simulink model "Transferfunction"  (R2021b)
settings: Solver=VariableStepAuto  StartTime=0.0  StopTime=10.0  RelTol=1e-3
libraries: dspsrcs4 x1
settings Model: Creator=Asus  LastModifiedBy=Matina Kaviani
settings SolverCC: AlgebraicLoopSolver=TrustRegion
settings DebuggingCC: SFMachineParentedDataDiag=warning

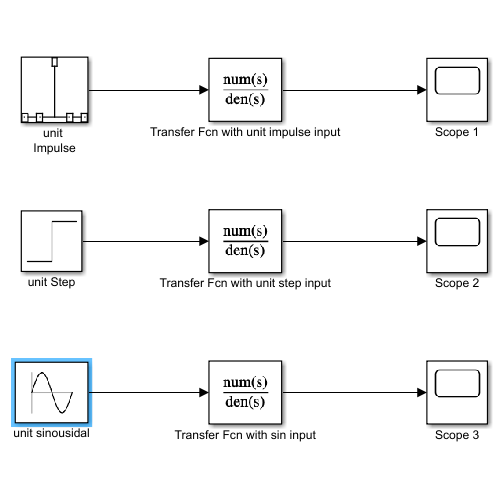
[thumbnail: Simulink's stored preview of the top-level diagram]
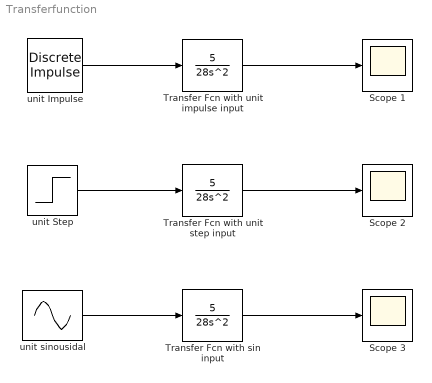
== system Transferfunction ==
  Scope 1 : Scope
  Scope 2 : Scope
  Scope 3 : Scope
  Transfer Fcn with sin input : TransferFcn  Numerator=[5]  Denominator=[28 0 0]
  Transfer Fcn with unit impulse input : TransferFcn  Numerator=[5]  Denominator=[28 0 0]
  Transfer Fcn with unit step input : TransferFcn  Numerator=[5]  Denominator=[28 0 0]
  unit Impulse : dspsrcs4/Discrete  Impulse  Delay=0  SampleTime=1  FrameSample=1  OutputFrames=off  dataType=double  isSigned=on  wordLen=16  udDataType=sfix(16)  fracBitsMode=Best precision  numFracBits=15  OutDataTypeStr=double  LastOutDataTypeStr=double
  unit Step : Step  SampleTime=0
  unit sinousidal : Sin  Frequency=2*pi  SampleTime=0
  wires:
  unit Step/1 -> Transfer Fcn with unit step input/1
  Transfer Fcn with unit step input/1 -> Scope 2/1
  unit sinousidal/1 -> Transfer Fcn with sin input/1
  Transfer Fcn with sin input/1 -> Scope 3/1
  unit Impulse/1 -> Transfer Fcn with unit impulse input/1
  Transfer Fcn with unit impulse input/1 -> Scope 1/1
